simulink model "demo_model"  (R2020b)
settings: Solver=FixedStepAuto  StartTime=0.0  StopTime=inf  RelTol=1e-3
libraries: DSX_Lib x7
settings Model: Creator=16047  LastModifiedBy=16047

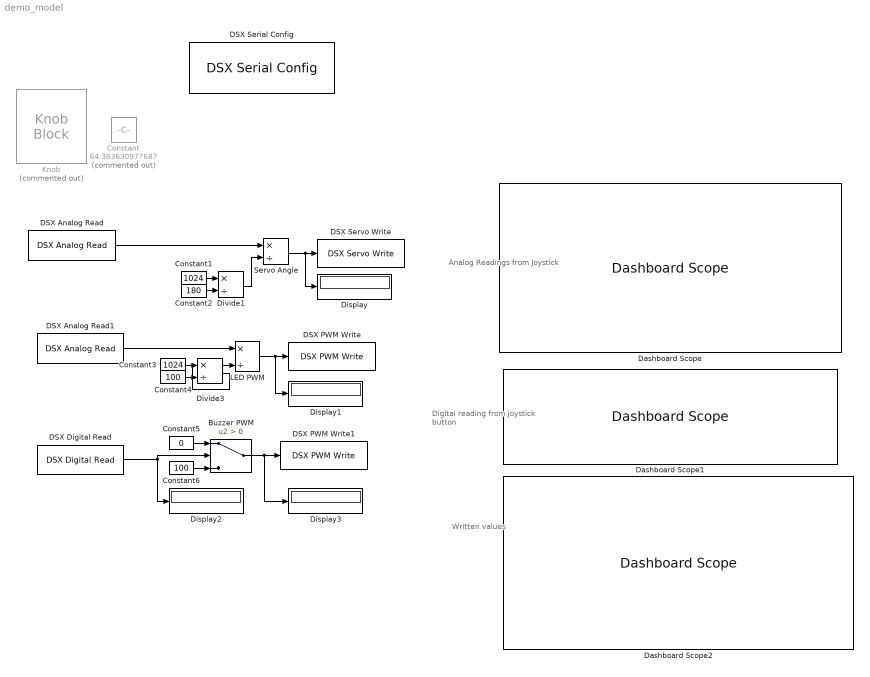
== system demo_model ==
  note: Analog Readings from Joystick
  note: Digital reading from joystick button
  note: Written values
  Buzzer PWM : Switch  Criteria=u2 > Threshold
  Constant : Constant  Commented=on  Value=64.363630977687
  Constant1 : Constant  Value=1024
  Constant2 : Constant  Value=180
  Constant3 : Constant  Value=1024
  Constant4 : Constant  Value=100
  Constant5 : Constant  Value=0
  Constant6 : Constant  Value=100
  DSX Analog Read : DSX_Lib/DSX Blocks/DSX Analog Read  aread_pin=A0
      settings: SourceProductName=DSX Library
  DSX Analog Read1 : DSX_Lib/DSX Blocks/DSX Analog Read  aread_pin=A1
      settings: SourceProductName=DSX Library
  DSX Digital Read : DSX_Lib/DSX Blocks/DSX Digital Read  read_pin=4
      settings: SourceProductName=DSX Library
  DSX PWM Write : DSX_Lib/DSX Blocks/DSX PWM Write  pwm_pin=3  pwm_freq=30
      settings: SourceProductName=DSX Library
  DSX PWM Write1 : DSX_Lib/DSX Blocks/DSX PWM Write  pwm_pin=5  pwm_freq=980
      settings: SourceProductName=DSX Library
  DSX Serial Config : DSX_Lib/DSX Blocks/DSX Serial Config  BaudRate=115200
      settings: SourceProductName=DSX Library
  DSX Servo Write : DSX_Lib/DSX Blocks/DSX Servo Write  servo_pin=6
      settings: SourceProductName=DSX Library
  Dashboard Scope : DashboardScope  Ymin=0  Ymax=1024
  Dashboard Scope1 : DashboardScope  Ymin=0  Ymax=1.1
  Dashboard Scope2 : DashboardScope  Ymin=0  Ymax=185
  Display{,1..3} (4 alike) : Display
  Divide1 : Product  Inputs=*/
  Divide3 : Product  Inputs=*/
  Knob : KnobBlock  Commented=on  ScaleMax=180
  LED PWM : Product  Inputs=*/
  Servo Angle : Product  Inputs=*/
  wires:
  DSX Analog Read/1 -> Servo Angle/1
  DSX Analog Read1/1 -> LED PWM/1
  Constant1/1 -> Divide1/1
  Constant2/1 -> Divide1/2
  Divide1/1 -> Servo Angle/2
  Servo Angle/1 -> Display/1, DSX Servo Write/1
  Divide3/1 -> LED PWM/2
  Constant4/1 -> Divide3/2
  Constant3/1 -> Divide3/1
  LED PWM/1 -> Display1/1, DSX PWM Write/1
  DSX Digital Read/1 -> Buzzer PWM/2, Display2/1
  Buzzer PWM/1 -> Display3/1, DSX PWM Write1/1
  Constant5/1 -> Buzzer PWM/1
  Constant6/1 -> Buzzer PWM/3
